simulink model "RPEM_FINAL"  (Simulink 5.0)
settings: Solver=ode45  StartTime=0.0  StopTime=10  RelTol=1e-3
undefined symbols (not defined in the file): ts
libraries: simulink x7, dspmtrx3 x3, dsparch4 x1
CloseFcn:
  | rtwprivate ssgensfun ModelCloseRequest rls
settings Model: LastModifiedBy=LeO

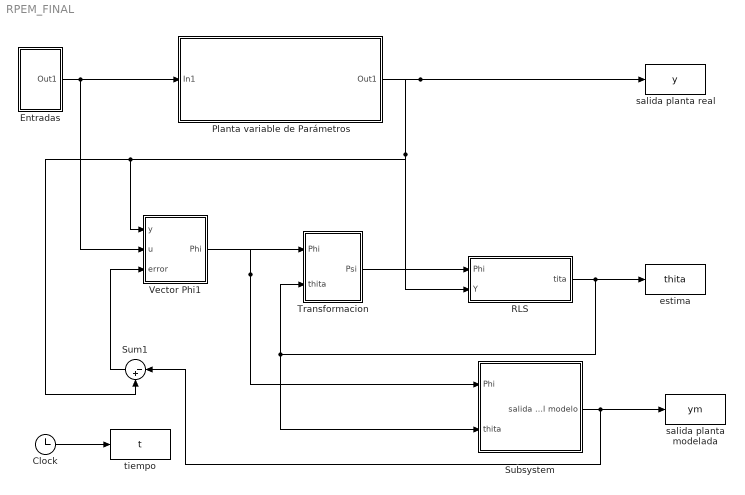
== system RPEM_FINAL ==
  Clock : Clock
      settings: Decimation=10
  Entradas : Subsystem
  Planta variable de Parámetros : Subsystem  mask{ruido=1, tiempo1=40}
      mask prompts: tiempo1 "tiempo de movimiento de parametros de la planta"
  RLS : Subsystem  mask{landa=0.1}
      mask prompts: landa "landa (factor de olvido)"
  Subsystem : Subsystem
  Sum1 : Sum  Orientation=left  Inputs=|-+  SaturateOnIntegerOverflow=on
  Transformacion : Subsystem
  Vector Phi1 : Subsystem  mask{nu=2, ny=3, ne=1, nk=1}
      mask prompts: nu "Nº de u tomadas"; ny "Nº de y tomadas"; ne "Nº de errores tomados"; nk "Nº de retardo"
  estima : ToWorkspace  VariableName=thita  SampleTime=ts  SaveFormat=Array
  salida planta modelada : ToWorkspace  VariableName=ym  SampleTime=ts  SaveFormat=Array
  salida planta real : ToWorkspace  VariableName=y  SampleTime=ts  SaveFormat=Array
  "tiempo " : ToWorkspace  VariableName=t  SampleTime=ts  SaveFormat=Array
  wires:
  Entradas/1(Out1) -> Planta variable de Parámetros/1(In1), Vector Phi1/2(u)
  Clock/1 -> "tiempo "/1
  Planta variable de Parámetros/1(Out1) -> salida planta real/1, Vector Phi1/1("y "), Sum1/2, RLS/2(Y)
  RLS/1(tita) -> estima/1, Subsystem/2(thita), Transformacion/2(thita)
  Vector Phi1/1(Phi) -> Subsystem/1(Phi), Transformacion/1(Phi)
  Subsystem/1(salida del modelo) -> salida planta modelada/1, Sum1/1
  Sum1/1 -> Vector Phi1/3(error)
  Transformacion/1(Psi) -> RLS/1("Phi ")

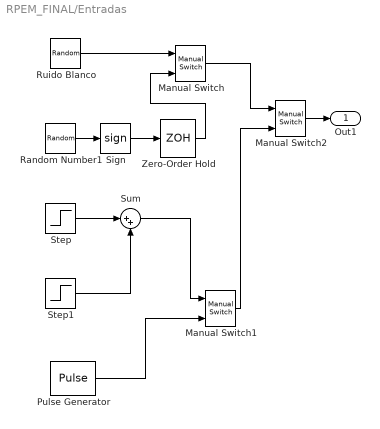
== system RPEM_FINAL/Entradas ==
  Manual Switch : simulink/Signal Routing/Manual Switch  sw=1  action=0
  Manual Switch1 : simulink/Signal Routing/Manual Switch  sw=1  action=0
  Manual Switch2 : simulink/Signal Routing/Manual Switch  sw=1  action=0
  Pulse Generator : DiscretePulseGenerator  PulseType=Time based  PulseWidth=50
  Random Number1 : RandomNumber  SampleTime=0
  Ruido Blanco : RandomNumber  Variance=20  Seed=12  SampleTime=ts
  Sign : Signum
  Step : Step  Time=2  After=2  SampleTime=0.05
  Step1 : Step  Time=50  After=5  SampleTime=0.05
  Sum : Sum  Inputs=|++  SaturateOnIntegerOverflow=on
  Zero-Order Hold : ZeroOrderHold  SampleTime=0.05
  Out1 : Outport
  wires:
  Sign/1 -> Zero-Order Hold/1
  Random Number1/1 -> Sign/1
  Manual Switch/1 -> Manual Switch2/1
  Ruido Blanco/1 -> Manual Switch/1
  Zero-Order Hold/1 -> Manual Switch/2
  Manual Switch2/1 -> Out1/1
  Step/1 -> Sum/1
  Step1/1 -> Sum/2
  Manual Switch1/1 -> Manual Switch2/2
  Sum/1 -> Manual Switch1/1
  Pulse Generator/1 -> Manual Switch1/2

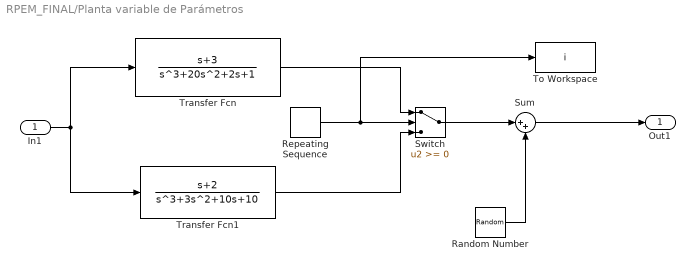
== system RPEM_FINAL/Planta variable de Parámetros ==
  In1 : Inport
  Random Number : RandomNumber  Variance=ruido  SampleTime=0
  Repeating Sequence : simulink/Sources/Repeating Sequence  rep_seq_t=[0 2*tiempo1]  rep_seq_y=[1 -1 ]
  Sum : Sum  Inputs=|++  SaturateOnIntegerOverflow=on
  Switch : Switch  SaturateOnIntegerOverflow=on
  To Workspace : ToWorkspace  VariableName=i  SampleTime=-1  SaveFormat=Array
  Transfer Fcn : TransferFcn  Numerator=[1 3 ]  Denominator=[1 20 2 1]
  Transfer Fcn1 : TransferFcn  Numerator=[1 2]  Denominator=[1 3 10 10]
  Out1 : Outport
  wires:
  Transfer Fcn/1 -> Switch/1
  Repeating Sequence/1 -> Switch/2, To Workspace/1
  Transfer Fcn1/1 -> Switch/3
  In1/1 -> Transfer Fcn/1, Transfer Fcn1/1
  Switch/1 -> Sum/1
  Sum/1 -> Out1/1
  Random Number/1 -> Sum/2

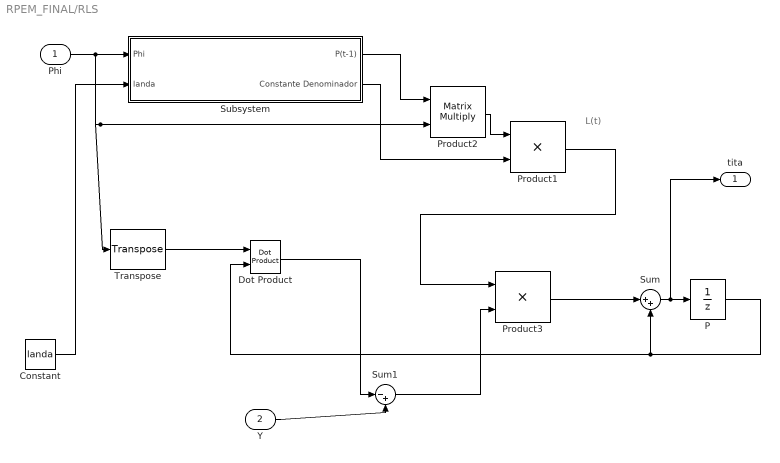
== system RPEM_FINAL/RLS ==
  note: L(t)
  "Phi " : Inport  SampleTime=ts
  Y : Inport  Port=2  SampleTime=ts
  Constant : Constant  Value=landa
  Dot Product : simulink/Math Operations/Dot Product
  P : UnitDelay  X0=10^-3  SampleTime=ts
  Product1 : Product  SaturateOnIntegerOverflow=on
  Product2 : Product  Multiplication=Matrix(*)  SaturateOnIntegerOverflow=on
  Product3 : Product  SaturateOnIntegerOverflow=on
  Subsystem : Subsystem
  Sum : Sum  Inputs=|++  SaturateOnIntegerOverflow=on
  Sum1 : Sum  Inputs=|-+  SaturateOnIntegerOverflow=on
  Transpose : dspmtrx3/Transpose  Hermitian=off
  tita : Outport
  wires:
  "Phi "/1 -> Subsystem/1(Phi), Product2/2, Transpose/1
  Constant/1 -> Subsystem/2(landa)
  Subsystem/1(P(t-1)) -> Product2/1
  Subsystem/2(Constante Denominador) -> Product1/2
  Product2/1 -> Product1/1
  Product1/1 -> Product3/1
  Sum/1 -> P/1, tita/1
  P/1 -> Sum/2, Dot Product/2
  Transpose/1 -> Dot Product/1
  Dot Product/1 -> Sum1/1
  Y/1 -> Sum1/2
  Sum1/1 -> Product3/2
  Product3/1 -> Sum/1

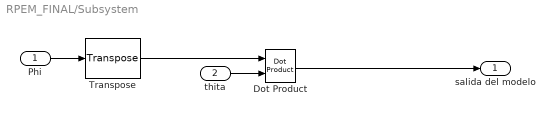
== system RPEM_FINAL/Subsystem ==
  Phi : Inport
  thita : Inport  Port=2
  Dot Product : simulink/Math Operations/Dot Product
  Transpose : dspmtrx3/Transpose  Hermitian=off
  salida del modelo : Outport
  wires:
  Transpose/1 -> Dot Product/1
  Phi/1 -> Transpose/1
  thita/1 -> Dot Product/2
  Dot Product/1 -> salida del modelo/1

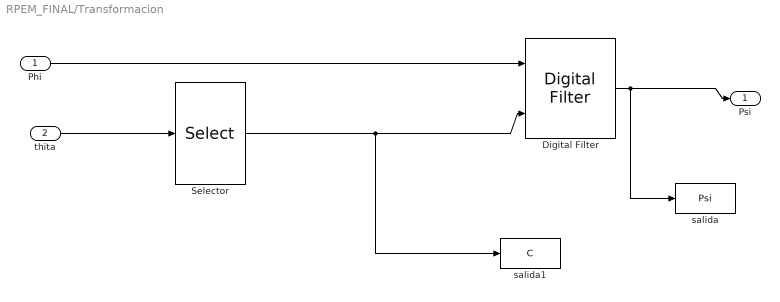
== system RPEM_FINAL/Transformacion ==
  Phi : Inport  SampleTime=ts
  thita : Inport  Port=2  SampleTime=ts
  Digital Filter : dsparch4/Digital Filter  TypePopup=IIR (all poles)  IIRFiltStruct=Direct form II transposed  AllPoleFiltStruct=Direct form  FIRFiltStruct=Direct form  CoeffSource=Input port(s)  NumCoeffs=[1 2]  DenCoeffs=[1 0.1]  BiQuadCoeffs=[1 0.3 0.4 1 0.1 0.2]  LatticeCoeffs=[0.2 0.4]  denIgnore=on  FiltPerSampPopup=One filter per sample  IC=0  ICnum=0  ICden=0
  Selector : Selector  Elements=[6]  InputPortWidth=6
  salida : ToWorkspace  VariableName=Psi  SampleTime=ts  SaveFormat=Array
  salida1 : ToWorkspace  VariableName=C  SampleTime=ts  SaveFormat=Array
  Psi : Outport
  wires:
  Phi/1 -> Digital Filter/1
  Digital Filter/1 -> salida/1, Psi/1
  thita/1 -> Selector/1
  Selector/1 -> salida1/1, Digital Filter/2

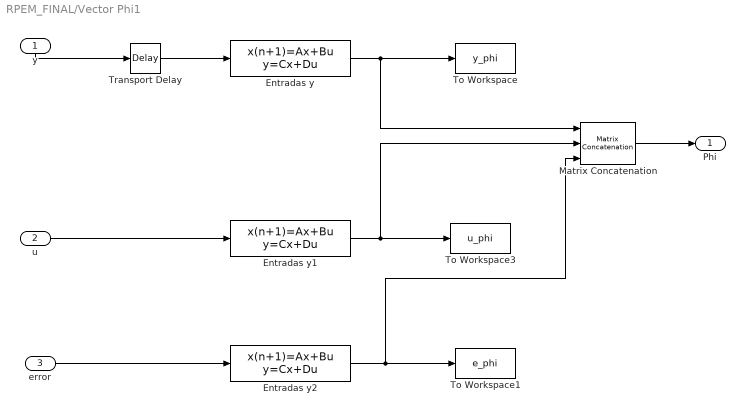
== system RPEM_FINAL/Vector Phi1 ==
  "y " : Inport  Orientation=down  SampleTime=ts
  u : Inport  Port=2  SampleTime=ts
  error : Inport  Port=3  SampleTime=ts
  Entradas y : DiscreteStateSpace  A=[zeros(1,ny) ;eye(ny-1,ny)]  B=[[-1 zeros(1,ny-1)]']  C=[eye(ny)]  D=[zeros(1,ny)']  SampleTime=ts
  Entradas y1 : DiscreteStateSpace  A=[zeros(1,nu) ;eye(nu-1,nu)]  B=[[-1 zeros(1,nu-1)]']  C=[eye(nu)]  D=[zeros(1,nu)']  SampleTime=ts
  Entradas y2 : DiscreteStateSpace  A=[zeros(1,ne) ;eye(ne-1,ne)]  B=[[-1 zeros(1,ne-1)]']  C=[eye(ne)]  D=[zeros(1,ne)']  SampleTime=ts
  Matrix Concatenation : simulink/Math Operations/Matrix Concatenation  numInports=3  catMethod=Vertical
  To Workspace : ToWorkspace  VariableName=y_phi  SampleTime=ts  SaveFormat=Array
  To Workspace1 : ToWorkspace  VariableName=e_phi  SampleTime=ts  SaveFormat=Array
  To Workspace3 : ToWorkspace  VariableName=u_phi  SampleTime=ts  SaveFormat=Array
  Transport Delay : TransportDelay  DelayTime=nk*ts
  Phi : Outport
  wires:
  "y "/1 -> Transport Delay/1
  u/1 -> Entradas y1/1
  Entradas y/1 -> To Workspace/1, Matrix Concatenation/1
  Entradas y1/1 -> To Workspace3/1, Matrix Concatenation/2
  Matrix Concatenation/1 -> Phi/1
  Transport Delay/1 -> Entradas y/1
  error/1 -> Entradas y2/1
  Entradas y2/1 -> To Workspace1/1, Matrix Concatenation/3

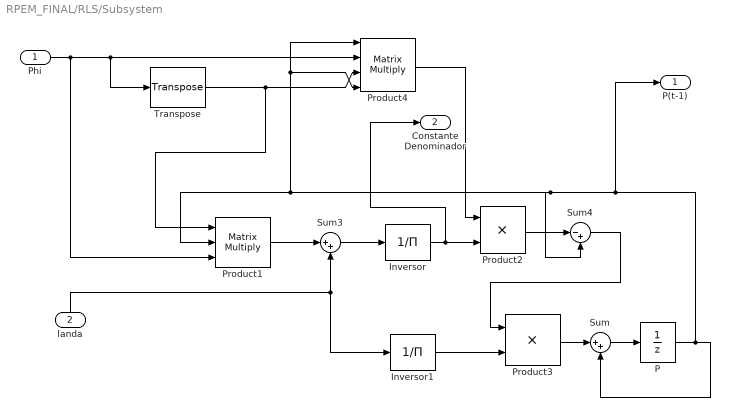
== system RPEM_FINAL/RLS/Subsystem ==
  Phi : Inport
  landa : Inport  Orientation=up  Port=2
  Inversor : Product  Inputs=/  SaturateOnIntegerOverflow=on
  Inversor1 : Product  Inputs=/  SaturateOnIntegerOverflow=on
  P : UnitDelay  X0=10^-3  SampleTime=ts
  Product1 : Product  Inputs=3  Multiplication=Matrix(*)  SaturateOnIntegerOverflow=on
  Product2 : Product  SaturateOnIntegerOverflow=on
  Product3 : Product  SaturateOnIntegerOverflow=on
  Product4 : Product  Inputs=4  Multiplication=Matrix(*)  SaturateOnIntegerOverflow=on
  Sum : Sum  Inputs=|++  SaturateOnIntegerOverflow=on
  Sum3 : Sum  Inputs=|++  SaturateOnIntegerOverflow=on
  Sum4 : Sum  Inputs=|-+  SaturateOnIntegerOverflow=on
  Transpose : dspmtrx3/Transpose  Hermitian=off
  P(t-1) : Outport
  Constante Denominador : Outport  Port=2
  wires:
  Phi/1 -> Product4/2, Transpose/1, Product1/3
  landa/1 -> Inversor1/1, Sum3/2
  Product4/1 -> Product2/1
  Inversor1/1 -> Product3/2
  Product3/1 -> Sum/1
  Inversor/1 -> Product2/2, Constante Denominador/1
  Sum3/1 -> Inversor/1
  Sum/1 -> P/1
  P/1 -> Sum/2, Sum4/2, Product1/2, Product4/1, Product4/4, P(t-1)/1
  Product1/1 -> Sum3/1
  Transpose/1 -> Product1/1, Product4/3
  Product2/1 -> Sum4/1
  Sum4/1 -> Product3/1
